simulink model "MRAC_simulation"  (R2018a)
settings: Solver=VariableStepAuto  StartTime=0.0  StopTime=100  RelTol=1e-3
values from neighbouring files (symbols this model uses):
  dyn_den = [1 20 56]    [MRAC_test.m]
  dyn_num = [18]    [MRAC_test.m]
  gam_p = 5    [MRAC_test.m]
  gam_pcmd = .1    (= 0.1)    [MRAC_test.m]
  ref_den = [coef_a coef_b coef_c]    [MRAC_test.m]
  ref_num = [coef_c]    [MRAC_test.m]
settings Model: Creator=ctf365  LastModifiedBy=ctf365

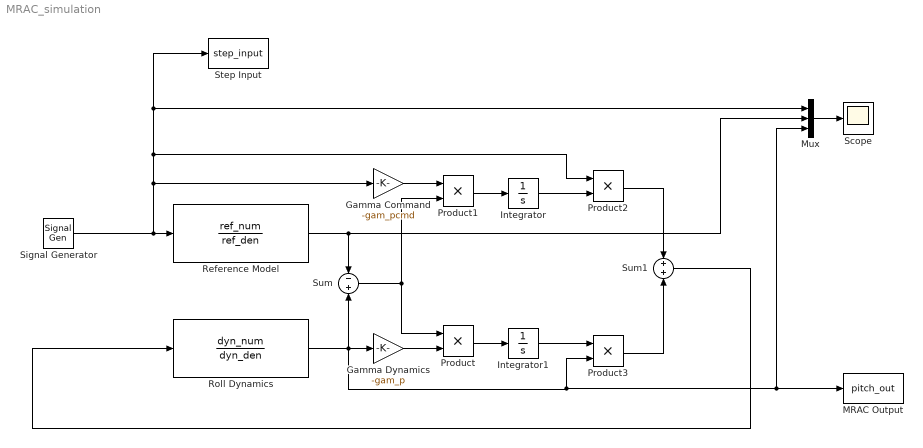
== system MRAC_simulation ==
  Gamma Command : Gain  Gain=-gam_pcmd
  Gamma Dynamics : Gain  Gain=-gam_p
  Integrator : Integrator
  Integrator1 : Integrator
  MRAC Output : ToWorkspace  VariableName=pitch_out  SaveFormat=Timeseries  SampleTime=-1
  Mux : Mux  Inputs=3
  Product{,1..3} (4 alike) : Product
  Reference Model : TransferFcn  Numerator=ref_num  Denominator=ref_den
  Roll Dynamics : TransferFcn  Numerator=dyn_num  Denominator=dyn_den
  Scope : Scope
  Signal Generator : SignalGenerator  WaveForm=square  Amplitude=20  Frequency=.2
  Step Input : ToWorkspace  VariableName=step_input  SaveFormat=Timeseries  SampleTime=-1
  Sum : Sum  Inputs=-+
  Sum1 : Sum
  wires:
  Reference Model/1 -> Sum/1, Mux/2
  Sum/1 -> Product/1, Product1/2
  Gamma Dynamics/1 -> Product/2
  Gamma Command/1 -> Product1/1
  Product/1 -> Integrator1/1
  Product1/1 -> Integrator/1
  Integrator/1 -> Product2/2
  Roll Dynamics/1 -> Sum/2, Gamma Dynamics/1, Mux/3, MRAC Output/1, Product3/2
  Integrator1/1 -> Product3/1
  Product2/1 -> Sum1/1
  Product3/1 -> Sum1/2
  Sum1/1 -> Roll Dynamics/1
  Signal Generator/1 -> Mux/1, Step Input/1, Product2/1, Gamma Command/1, Reference Model/1
  Mux/1 -> Scope/1
